simulink model "sputnik"  (R2021b)
settings: Solver=VariableStepAuto  StartTime=0.0  StopTime=1000.0  FixedStep=1e-3  MaxStep=0.1  RelTol=1e-3
libraries: matrix_library x1
settings Model: Creator=Mslv  LastModifiedBy=Mslv

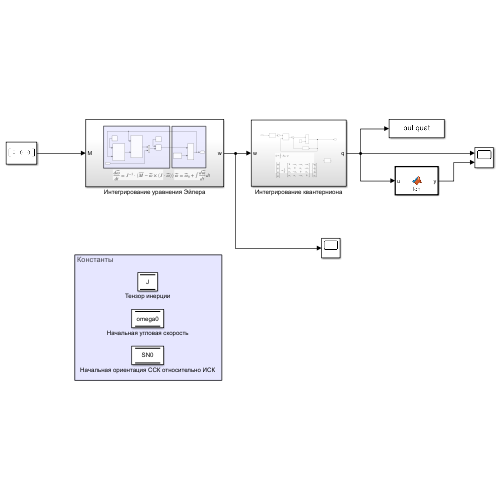
[thumbnail: Simulink's stored preview of the top-level diagram]
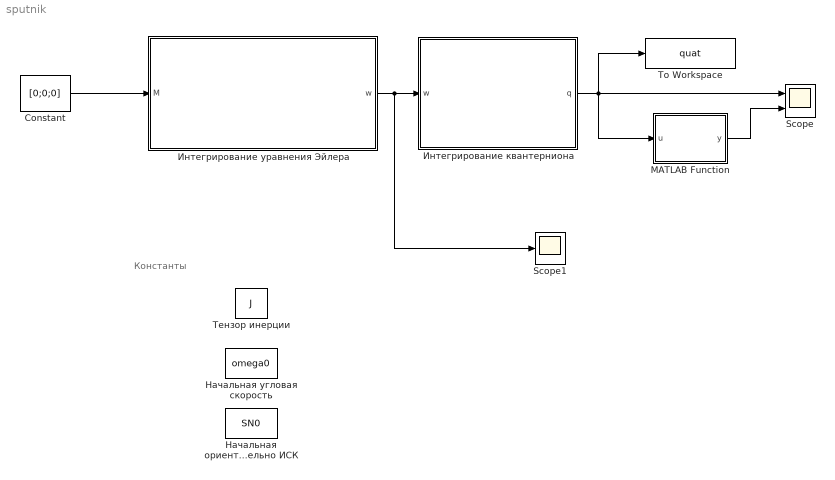
== system sputnik ==
  note: Константы
  Constant : Constant  Value=[0;0;0]
  MATLAB Function : MATLAB Function  TreatAsAtomicUnit=on
  Scope : Scope  NumInputPorts=2
  Scope1 : Scope
  To Workspace : ToWorkspace  VariableName=quat  SampleTime=-1
  Интегрирование квантерниона : Subsystem
  Интегрирование уравнения Эйлера : Subsystem
  Начальная ориентация ССК относительно ИСК : DataStoreMemory  DataStoreName=SN0  InitialValue=[1;0;0;0]  ShowAdditionalParam=off
  Начальная угловая скорость : DataStoreMemory  DataStoreName=omega0  InitialValue=[0;0;0.003]  ShowAdditionalParam=off
  Тензор инерции : DataStoreMemory  DataStoreName=J  InitialValue=[2416.66666666667 0 0;0 2237.5 0;0 0 2179.16666666667]  ShowAdditionalParam=off
  wires:
  Constant/1 -> Интегрирование уравнения Эйлера/1(M)
  Интегрирование уравнения Эйлера/1(w) -> Scope1/1, Интегрирование квантерниона/1(w)
  Интегрирование квантерниона/1(q) -> MATLAB Function/1(u), To Workspace/1, Scope/1
  MATLAB Function/1(y) -> Scope/2

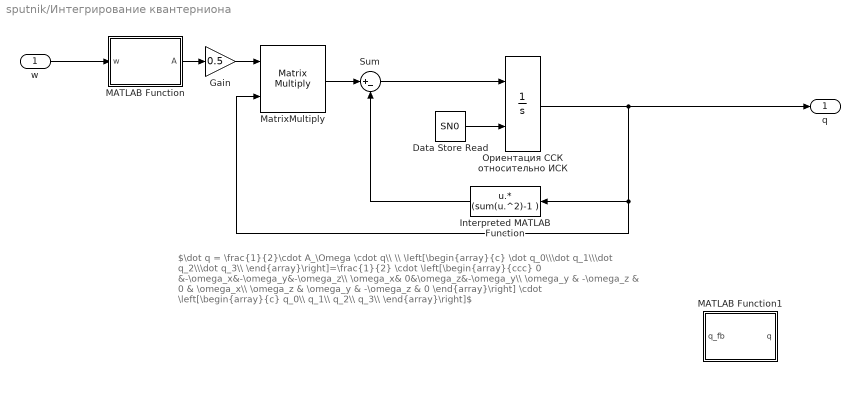
== system sputnik/Интегрирование квантерниона ==
  note: $\dot q = \frac{1}{2}\cdot A_\Omega \cdot q\\ \\ \left[\begin{array}{c} \dot q_0\\\dot q_1\\\dot q_2\\\dot q_3\\ \end{array}\right]=\frac{1}{2} \cdot \left[\begin{array}{ccc} 0 &-\omega_x&-\omega_y&-\omega_z\\ \omega_x& 0&\omega_z&-\omega_y\\ \omega_y & -\omega_z & 0 & \omega_x\\ \omega_z & \omega_y & -\omega_z & 0 \end{array}\right] \cdot \left[\begin{array}{c} q_0\\ q_1\\ q_2\\ q_3\\ \end{array}\right]$
  w : Inport
  Data Store Read : DataStoreRead  DataStoreName=SN0  IndexOptions=Index vector (dialog)  Indices=1  OutputSizes=1
  Gain : Gain  Gain=0.5
  Interpreted MATLAB Function : MATLABFcn  MATLABFcn=u.* (sum(u.^2)-1 )  OutputDimensions=[4,1]  Output1D=off
  MATLAB Function : MATLAB Function  TreatAsAtomicUnit=on
  MATLAB Function1 : MATLAB Function  TreatAsAtomicUnit=on
  MatrixMultiply : Product  Multiplication=Matrix(*)
  Sum : Sum  Inputs=|+-
  Ориентация ССК относительно ИСК : Integrator  InitialConditionSource=external
  q : Outport
  wires:
  Data Store Read/1 -> Ориентация ССК относительно ИСК/2
  w/1 -> MATLAB Function/1(w)
  MATLAB Function/1(A) -> Gain/1
  Gain/1 -> MatrixMultiply/1
  MatrixMultiply/1 -> Sum/1
  Sum/1 -> Ориентация ССК относительно ИСК/1
  Interpreted MATLAB Function/1 -> Sum/2
  Ориентация ССК относительно ИСК/1 -> q/1, Interpreted MATLAB Function/1, MatrixMultiply/2

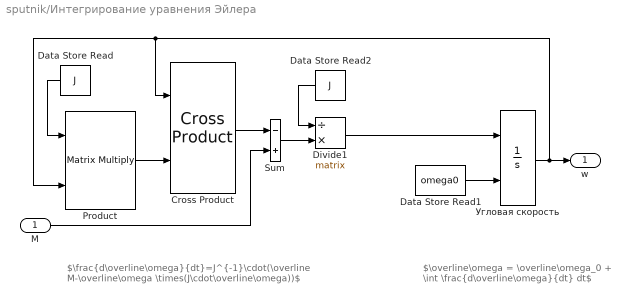
== system sputnik/Интегрирование уравнения Эйлера ==
  note: $\frac{d\overline\omega}{dt}=J^{-1}\cdot(\overline M-\overline\omega \times(J\cdot\overline\omega))$
  note: $\overline\omega = \overline\omega_0 + \int \frac{d\overline\omega}{dt} dt$
  M : Inport
  Cross Product : matrix_library/Cross Product
      settings: SourceProductBaseCode=SL
  Data Store Read : DataStoreRead  DataStoreName=J  IndexOptions=Index vector (dialog)  Indices=1  OutputSizes=1
  Data Store Read1 : DataStoreRead  DataStoreName=omega0  IndexOptions=Index vector (dialog)  Indices=1  OutputSizes=1
  Data Store Read2 : DataStoreRead  DataStoreName=J  IndexOptions=Index vector (dialog)  Indices=1  OutputSizes=1
  Divide1 : Product  Inputs=/*  Multiplication=Matrix(*)
  Product : Product  Inputs=**  Multiplication=Matrix(*)
  Sum : Sum  Inputs=-+
  Угловая скорость : Integrator  InitialConditionSource=external
  w : Outport
  wires:
  M/1 -> Sum/2
  Sum/1 -> Divide1/2
  Угловая скорость/1 -> w/1, Product/2, Cross Product/1
  Cross Product/1 -> Sum/1
  Data Store Read1/1 -> Угловая скорость/2
  Divide1/1 -> Угловая скорость/1
  Data Store Read/1 -> Product/1
  Product/1 -> Cross Product/2
  Data Store Read2/1 -> Divide1/1

== matlab function sputnik/Интегрирование квантерниона/MATLAB Function ==
  data: w input; A output
function A = omegaMatrix(w)

A=[
    0    -w(1) -w(2) -w(3)
    w(1)  0     w(3) -w(2)
    w(2) -w(3)  0     w(1)
    w(3)  w(2) -w(1)  0
    ];

== matlab function sputnik/MATLAB Function ==
  data: u input; y output
function y = fcn(u)

y = sum(u.^2);

== matlab function sputnik/Интегрирование квантерниона/MATLAB Function1 ==
  data: q input; q_fb output
function q_fb = fcn(q)
q_fb = q.* (sum(q.^2)-1 );
